simulink model "controlled_model"  (R2015b)
settings: Solver=VariableStepAuto  StartTime=0.0  StopTime=10.0  RelTol=1e-3
settings Model: Creator=yuji  LastModifiedBy=yuji

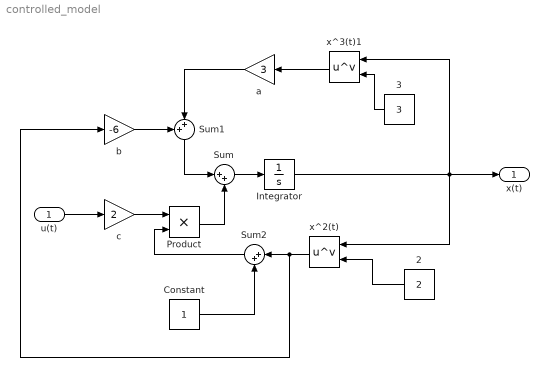
== system controlled_model ==
  u(t) : Inport
  2 : Constant  Value=2
  3 : Constant  Value=3
  Constant : Constant
  Integrator : Integrator
  Product : Product
  Sum : Sum  Inputs=|++
  Sum1 : Sum  Inputs=++|
  Sum2 : Sum  Inputs=|++
  a : Gain  Gain=3
  b : Gain  Gain=-6
  c : Gain  Gain=2
  x^2(t) : Math  Operator=pow  SaturateOnIntegerOverflow=on
  x^3(t)1 : Math  Operator=pow  SaturateOnIntegerOverflow=on
  x(t) : Outport
  wires:
  u(t)/1 -> c/1
  Integrator/1 -> x^2(t)/1, x^3(t)1/1, x(t)/1
  2/1 -> x^2(t)/2
  3/1 -> x^3(t)1/2
  Sum/1 -> Integrator/1
  Product/1 -> Sum/2
  c/1 -> Product/1
  Sum1/1 -> Sum/1
  b/1 -> Sum1/1
  x^2(t)/1 -> b/1, Sum2/1
  Sum2/1 -> Product/2
  x^3(t)1/1 -> a/1
  a/1 -> Sum1/2
  Constant/1 -> Sum2/2
